simulink model "HANcoder_Olimexino_F3"  (R2018b)
settings: Solver=FixedStepDiscrete  StartTime=0.0  StopTime=2  FixedStep=0.01  RelTol=1e-3
PreLoadFcn:
  | librarySetup
  | eval([bdroot,'_startup']) %Calling [modelName]_startup.m
undefined symbols (not defined in the file or in its folder): A0, A1, A2, A3, A4, A5, CON2, CON3, CON4, D0, D14, D2, D24, D3, D5, D9, EXT, F3, HANtuneOverride, LED2, pwm, TIM2, TIM4, USB
libraries: HANcoder_STM32_Target x25, simulink x2
CloseFcn:
  | rtwprivate ssgencode ModelCloseRequest mytest
settings Model: Creator=Jason van Kolfschoten  LastModifiedBy=rickg
settings SolverCC: PositivePriorityOrder=on
settings DataIOCC: LimitDataPoints=on  SaveFormat=Array  SignalLoggingSaveFormat=ModelDataLogs  SaveOutput=off  SaveTime=off
settings OptimizationCC: BlockReduction=off  DefaultParameterBehavior=Inlined  DefaultUnderspecifiedDataType=single  InlineInvariantSignals=on  ExpressionDepthLimit=2147483647  StateBitsets=on  DataBitsets=on  ZeroExternalMemoryAtStartup=off  ZeroInternalMemoryAtStartup=off  InitFltsAndDblsToZero=on  NoFixptDivByZeroProtection=on  EfficientFloat2IntCast=on  LifeSpan=inf
settings DebuggingCC: SaveWithDisabledLinksMsg=none  SaveWithParameterizedLinksMsg=none  CheckSSInitialOutputMsg=off  UnderspecifiedInitializationDetection=Classic  MergeDetectMultiDrivingBlocksExec=none  SignalResolutionControl=TryResolveAll  SolverPrmCheckMsg=warning  InheritedTsInSrcMsg=none  MultiTaskDSMMsg=warning  MultiTaskCondExecSysMsg=none  ParameterPrecisionLossMsg=none  FcnCallInpInsideContextMsg=warning  StateNameClashWarn=warning  SFUnexpectedBacktrackingDiag=warning  SFNoUnconditionalDefaultTransitionDiag=warning  SFExecutionAtInitializationDiag=none
settings HardwareCC: ProdBitPerPointer=32  ProdBitPerSizeT=32  ProdBitPerPtrDiffT=32  ProdLargestAtomicInteger=Long  ProdLargestAtomicFloat=Double  ProdWordSize=32  ProdHWDeviceType=ARM Compatible->ARM Cortex  TargetEndianess=LittleEndian  TargetHWDeviceType=Infineon->TriCore
settings ModelReferenceCC: PropagateSignalLabelsOutOfModel=off
settings SFSimCC: SimUseLocalCustomCode=off  MATLABDynamicMemAlloc=off
settings RTWCC: SystemTargetFile=ert.tlc  MakeCommand=make_rtw SHELL= HANcoder_PORTABLE=1 HANcoder_BOOTLOADER=1  TemplateMakefile=Olimexino_STM32_F3_gcc.tmf  Description=Real-Time Workshop Embedded Coder (no auto configuration)  RTWUseLocalCustomCode=off
settings CodeAppCC: ForceParamTrailComments=on  IgnoreCustomStorageClasses=off  SimulinkDataObjDesc=on  CustomSymbolStrGlobalVar=rt$N$M  CustomSymbolStrType=$N$M  CustomSymbolStrFcn=$N$M$F  CustomSymbolStrMacro=$N$M  InsertBlockDesc=on  StateflowObjectComments=on  InternalIdentifier=Classic
settings ERTTargetCC: TargetFcnLib=ansi_tfl_tmw.mat  MultiwordLength=2048  IncludeMdlTerminateFcn=off  SuppressErrorStatus=on  SupportNonFinite=off  GenerateASAP2=on  InlinedParameterPlacement=NonHierarchical  ERTCustomFileTemplate=example_file_process.tlc  ConvertIfToSwitch=off  SuppressUnreachableDefaultCases=off
settings ConfigComp: CovMetricSettings=dw  CovHtmlReporting=on  CovSaveCumulativeToWorkspaceVar=on  CovSaveSingleToWorkspaceVar=on  CovExternalEMLEnable=off  CovSFcnEnable=off  DVMaxProcessTime=600  DVDisplayUnsatisfiableObjectives=on  DVAutomaticStubbing=off  DVSubSystemToStub=7.76600366011452e-316  DVParameterNames=7.76600366011452e-316  DVParameterConstraints=7.76600366011452e-316  DVParameterUseInAnalysis=7.76600366011452e-316  DVModelCoverageObjectives=MCDC  DVMaxTestCaseSteps=500  DVTestSuiteOptimization=CombinedObjectives  DVDetectActiveLogic=on  DVSaveHarnessModel=on

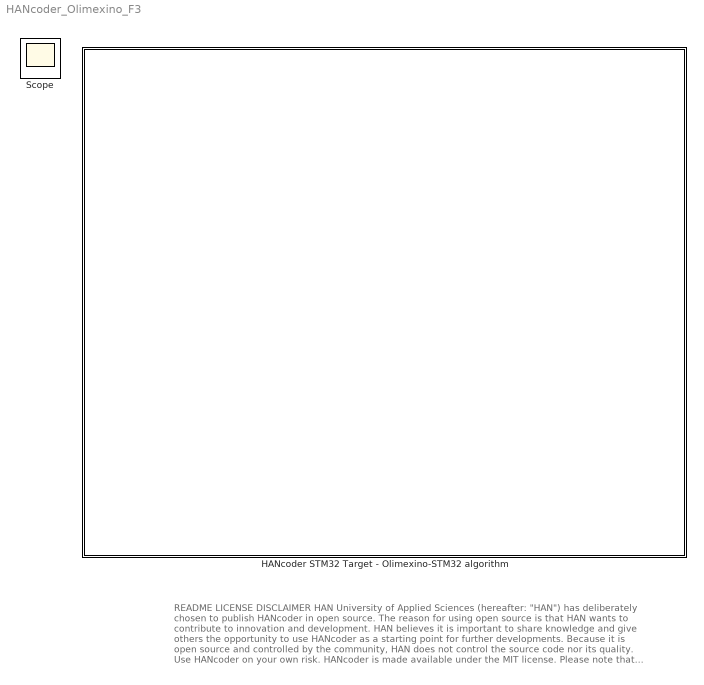
== system HANcoder_Olimexino_F3 ==
  note: README
      |
      | LICENSE
      |
      | DISCLAIMER
      |
      | HAN University of Applied Sciences (hereafter: "HAN") has deliberately chosen
      | to publish HANcoder in open source. The reason for using open source is that
      | HAN wants to contribute to innovation and development. HAN believes it is
      | important to share knowledge and give others the opportunity to use HANcoder
      | as a starting point for further developments. Because it is open source and
      | controlled by the community, HAN does not control the source code nor its
      | quality. Use HANcoder on your own risk. HANcoder is made available under the
      | MIT license. Please note that this license contains an exclusion of liability.
  HANcoder STM32 Target - Olimexino-STM32 algorithm : Subsystem  mask(TopLevelSubsystem){}
      mask Display: image(imread('Olimexino_STM32_HAN.jpg'))
  Scope : Scope

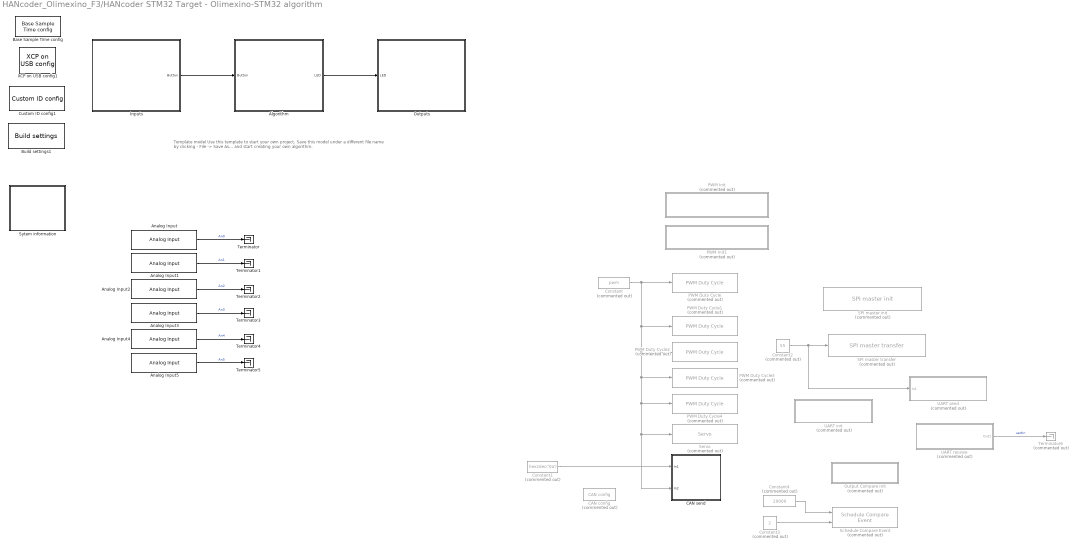
== system HANcoder_Olimexino_F3/HANcoder STM32 Target - Olimexino-STM32 algorithm ==
  note: Template model
      | Use this template to start your own project. Save this model
      | under a different file name by clicking - File -> Save As... and
      | start creating your own algorithm.
  Algorithm : Subsystem
  Analog Input : HANcoder_STM32_Target/Olimexino STM32 F3/Analog Inputs/Analog Input  Tag=HANcoder_TARGET_STM32_F3_Olimexino  pinID=CON2 - A0  tsamp=-1  filtered=off
      settings: SourceProductName=HANcoder STM32 Target
  Analog Input1 : HANcoder_STM32_Target/Olimexino STM32 F3/Analog Inputs/Analog Input  Tag=HANcoder_TARGET_STM32_F3_Olimexino  pinID=CON2 - A1  tsamp=-1  filtered=off
      settings: SourceProductName=HANcoder STM32 Target
  Analog Input2 : HANcoder_STM32_Target/Olimexino STM32 F3/Analog Inputs/Analog Input  Tag=HANcoder_TARGET_STM32_F3_Olimexino  pinID=CON2 - A2  tsamp=-1  filtered=off
      settings: SourceProductName=HANcoder STM32 Target
  Analog Input3 : HANcoder_STM32_Target/Olimexino STM32 F3/Analog Inputs/Analog Input  Tag=HANcoder_TARGET_STM32_F3_Olimexino  pinID=CON2 - A3  tsamp=-1  filtered=off
      settings: SourceProductName=HANcoder STM32 Target
  Analog Input4 : HANcoder_STM32_Target/Olimexino STM32 F3/Analog Inputs/Analog Input  Tag=HANcoder_TARGET_STM32_F3_Olimexino  pinID=CON2 - A4  tsamp=-1  filtered=off
      settings: SourceProductName=HANcoder STM32 Target
  Analog Input5 : HANcoder_STM32_Target/Olimexino STM32 F3/Analog Inputs/Analog Input  Tag=HANcoder_TARGET_STM32_F3_Olimexino  pinID=CON2 - A5  tsamp=-1  filtered=off
      settings: SourceProductName=HANcoder STM32 Target
  Base Sample Time config : HANcoder_STM32_Target/Olimexino STM32 F3/System Config/Base Sample Time config  Tag=HANcoder_TARGET_STM32_F3_Olimexino  Description=HANcoder Target STM32-Olimexino blockset version 1.2  baseSampleTime=10  extraStack=25
      settings: SourceProductName=HANcoder STM32 Target
  Build settings1 : HANcoder_STM32_Target/Olimexino STM32 F3/System Config/Build settings  Tag=HANcoder_TARGET_STM32_F3_Olimexino  AutoASAP2add=on  AutoFlash=USB-F3
      settings: SourceProductName=HANcoder STM32 Target
  CAN config : HANcoder_STM32_Target/Olimexino STM32 F3/System Config/CAN config  Tag=HANcoder_TARGET_STM32_F3_Olimexino  Commented=on  canBus1=on  baudRate1=250  rxMask1=hex2dec('00000000')  rxCode1=hex2dec('00000000')  rxMode1=Receive only 11-bit message identifiers  txBufSize1=32  evBufSize1=8
      settings: SourceProductName=HANcoder STM32 Target
  CAN send : Subsystem  Tag=HANcoder_TARGET_STM32_F3_Olimexino  AncestorBlock=HANcoder_STM32_Target/Olimexino STM32 F3/CAN/CAN/CAN send  mask(CAN send){canBus=CAN 1, frameType=Standard (11 bit), inputNumber=1, dataType=uint16, byteOrder=on, tsamp=0.1}
      mask prompts: canBus "CAN channel"; frameType "Identifier type"; inputNumber "Input ports"; dataType "Input datatype"; byteOrder "Byte order: Checked = MSB first, unchecked = LSB first."; tsamp "Sample time"
      mask help:
      | Function
      | ==========
      | Send a message on the CAN channel.
      |
      | Parameters
      | ==========
      | CAN channel:           The CAN channel to send the message on.
      | Identifier type:         normal or extended ID's
      | Input ports:              The amount of input ports
      | Input datatype:        The datatype of the input ports
      | Byte order:               Select MSB or LSB first
      | Sample time:            -1 or divisible by base sample time [seconds]
      |
      | Input
      | ==========
      | Port 1:                   CAN ID(uint32) in hexadecimal ie: hex2dec('0a')
      | Port 2..9                CAN message data
      mask init:
      | sfcn_can_send_mcb(canBus, frameType, inputNumber, dataType, byteOrder)
      settings: MoveFcn=drawLogos
      mask Help: web('sfcn_can_send.html');
      mask TypeOptions canBus: CAN 1
      mask TypeOptions frameType: Standard (11 bit) | Extended (29 bit)
      mask TypeOptions dataType: int8 | uint8 | int16 | uint16 | int32 | uint32 | boolean
      mask Display:
      | fprintf('Send on\nCAN %x', canBus);
      | port_label('input', 1, 'ID');patch([89 108 107 88],[2 6 10 6],[0.89804 0 0.33725]);
  Constant : Constant  Commented=on  Value=pwm  OutDataTypeStr=uint16
  Constant1 : Constant  Commented=on  Value=hex2dec('0a')  OutDataTypeStr=uint32
  Constant2 : Constant  Commented=on  Value=55  OutDataTypeStr=uint8
  Constant3 : Constant  Commented=on  Value=2  OutDataTypeStr=uint8
  Constant4 : Constant  Commented=on  Value=20000  OutDataTypeStr=uint16
  Custom ID config1 : HANcoder_STM32_Target/Olimexino STM32 F3/System Config/Custom ID config  Tag=HANcoder_TARGET_STM32_F3_Olimexino  softID=softwareID  softNUM=1
      settings: SourceProductName=HANcoder STM32 Target
  Inputs : Subsystem
  Output Compare Init : Subsystem  Tag=HANcoder_TARGET_STM32_F3_Olimexino  Commented=on  AncestorBlock=HANcoder_STM32_Target/Olimexino STM32 F3/Timer Outputs/Output Compare Init  mask(Output Compare Init){moduleID=TIM2: D2 & D3 & D1 & D0, frequency=2000000, enableIRQoutput=off}
      mask prompts: moduleID "Timer module"; frequency "Frequency (free running counter) [Hz]"; enableIRQoutput "Enable IRQ output"
      mask help:
      | Function
      | ========
      | Initializes the timer module to allow output compare functionality on the
      | module's channels.
      |
      | Parameters
      | ==========
      | Timer Module:
      |   Selects the timer module.
      |
      | Frequency:
      |   Frequency at which the 16-bit free running counter counts.
      |
      | Enable IRQ output
      |   Controls whether or not the IRQ output is available.
      |
      | Outport
      | =======
      | IRQ
      |   Allows connection of a function call subsystem for the free running
      |   counter overflow event.
      mask init:
      | moduleIDInfoStr = sfcn_timeout_init_mcb(1, moduleID, frequency, enableIRQoutput);
      settings: CopyFcn=sfcn_timeout_init_chk();  MoveFcn=drawLogos
      mask Help: web('sfcn_timeout_init.html');
      mask TypeOptions moduleID: TIM1: D6 & D7 & D8 & n/a | TIM2: D2 & D3 & D1 & D0 | TIM3: D35 & D36 & D37 & n/a | TIM4: D5 & D9 & D14 & D24
      mask Callback moduleID: sfcn_timeout_init_chk();
      mask Display: fprintf('Output Compare Init\n%s', moduleIDInfoStr);patch([129 148 147 128],[2 6 10 6],[0.89804 0 0.33725]);
  Outputs : Subsystem
  PWM Duty Cycle : HANcoder_STM32_Target/Olimexino STM32 F3/PWM Outputs/PWM Duty Cycle  Tag=HANcoder_TARGET_STM32_F3_Olimexino  Commented=on  pinID=TIM2 - CON3 - D0  tsamp=-1
      settings: SourceProductName=HANcoder STM32 Target
  PWM Duty Cycle1 : HANcoder_STM32_Target/Olimexino STM32 F3/PWM Outputs/PWM Duty Cycle  Tag=HANcoder_TARGET_STM32_F3_Olimexino  Commented=on  pinID=TIM4 - CON3 - D5  tsamp=-1
      settings: SourceProductName=HANcoder STM32 Target
  PWM Duty Cycle2 : HANcoder_STM32_Target/Olimexino STM32 F3/PWM Outputs/PWM Duty Cycle  Tag=HANcoder_TARGET_STM32_F3_Olimexino  Commented=on  pinID=TIM4 - CON4 - D9  tsamp=-1
      settings: SourceProductName=HANcoder STM32 Target
  PWM Duty Cycle3 : HANcoder_STM32_Target/Olimexino STM32 F3/PWM Outputs/PWM Duty Cycle  Tag=HANcoder_TARGET_STM32_F3_Olimexino  Commented=on  pinID=TIM4 - CON4 - D14  tsamp=-1
      settings: SourceProductName=HANcoder STM32 Target
  PWM Duty Cycle4 : HANcoder_STM32_Target/Olimexino STM32 F3/PWM Outputs/PWM Duty Cycle  Tag=HANcoder_TARGET_STM32_F3_Olimexino  Commented=on  pinID=TIM4 - EXT - D24  tsamp=-1
      settings: SourceProductName=HANcoder STM32 Target
  PWM Init : Subsystem  Tag=HANcoder_TARGET_STM32_F3_Olimexino  Commented=on  AncestorBlock=HANcoder_STM32_Target/Olimexino STM32 F3/PWM Outputs/PWM Init  mask(Pulse Width Modulation Initialization){moduleID=TIM2: D2 & D3 & n/a & D0, frequency=5022, alignment=Edge aligned, enableIRQoutput=off, ch1On=off, ch1Pol=Active high, ch1Inv=off, ch2On=off, ch2Pol=Active high, ch2Inv=off, ch3On=off, ch3Pol=Active high, ch3Inv=off, ch4On=on, ch4Pol=Active high, ch4Inv=off}
      mask prompts: moduleID "PWM module"; frequency "Signal frequency [Hz]"; alignment "Signal alignment"; enableIRQoutput "Enable IRQ output"; ch1On "Generate PWM signal on channel 1"; ch1Pol "Select signal polarity"; ch1Inv "Enable inverted signal on additional output pin"; ch2On "Generate PWM signal on channel 2"; ch2Pol "Select signal polarity"; ch2Inv "Enable inverted signal on additional output pin"; ch3On "Generate PWM signal on channel 3"; ch3Pol "Select signal polarity"; ch3Inv "Enable inverted signal on additional output pin"; ch4On "Generate PWM signal on channel 4"; ch4Pol "Select signal polarity"; ch4Inv "Enable inverted signal on additional output pin"
      mask help:
      | Function
      | ========
      | A 'PWM Init' block configures one of the STM32 timer modules for PWM
      | functionality, allowing a PWM signal to be generated on up to 4 timer
      | channels and their associated output pins.
      |
      | Parameters
      | ==========
      | General - PWM module:
      |   Select the PWM module to use. The name in the combo box contains
      |   information about which pins on the target belong to this timer module.
      |   Also the first pin corresponds with the first channel and so on:
      |   TIMx: Ch1 & Ch2 & Ch3...
      |
      | General - Signal frequency:
      |   Determines the signal frequency in Hz. If you click 'Apply' after entering
      |   the desired frequency it will automatically be adjusted to the closest
      |   supported value.
      |
      | General - Signal Aligment:
      |   Determines the aligment of the signal. It can either be edge aligned or
      |   center aligned.
      |
      | General - Enable IRQ output
      |   Controls whether or not the IRQ output is available.
      |
      | Channel x - Generate PWM signal on channel x:
      |   Enable to configure the channel for PWM functionality so that the PWM signal
      |   is outputted on the channel's associated microcontroller pin.
      |
      | Channel x - Signal polarity:
      |   Selects the polarity of the signal.
      |
      | Channel x - Enable inverted signal on additional output pin:
      |   When enabled, a second PWM signal will be generated on an additional
      |   microcontroller pin where the signal is an exact inversion of the first signal.
      mask init:
      | moduleIDInfoStr = sfcn_pwmout_init_mcb(1, moduleID, frequency, alignment, enableIRQoutput, ch1On, ch2On, ch3On, ch4On, ch1Pol, ch2Pol, ch3Pol, ch4Pol, ch1Inv, ch2Inv, ch3Inv, ch4Inv);
      settings: CopyFcn=sfcn_pwmout_init_chk();  MoveFcn=drawLogos
      mask Help: web('sfcn_pwmout_init.html');
      mask TypeOptions moduleID: TIM1: D6 & D7 & D8 & n/a + N-channels D32 & D33 & D34  | TIM2: D2 & D3 & n/a & D0 | TIM3: D35 & D36 & D37 & n/a | TIM4: D5 & D9 & D14 & D24
      mask Callback moduleID: sfcn_pwmout_init_chk();
      mask TypeOptions alignment: Edge aligned | Center aligned
      mask TypeOptions ch1Pol: Active high | Active low
      mask TypeOptions ch2Pol: Active high | Active low
      mask TypeOptions ch3Pol: Active high | Active low
      mask TypeOptions ch4Pol: Active high | Active low
      mask Display: fprintf('PWM Init\n%s', moduleIDInfoStr);patch([214 233 232 213],[2 6 10 6],[0.89804 0 0.33725]);
  PWM Init1 : Subsystem  Tag=HANcoder_TARGET_STM32_F3_Olimexino  Commented=on  AncestorBlock=HANcoder_STM32_Target/Olimexino STM32 F3/PWM Outputs/PWM Init  mask(Pulse Width Modulation Initialization){moduleID=TIM4: D5 & D9 & D14 & D24, frequency=5022, alignment=Edge aligned, enableIRQoutput=off, ch1On=on, ch1Pol=Active high, ch1Inv=off, ch2On=on, ch2Pol=Active high, ch2Inv=off, ch3On=off, ch3Pol=Active high, ch3Inv=off, ch4On=off, ch4Pol=Active high, ch4Inv=off}
      mask prompts: moduleID "PWM module"; frequency "Signal frequency [Hz]"; alignment "Signal alignment"; enableIRQoutput "Enable IRQ output"; ch1On "Generate PWM signal on channel 1"; ch1Pol "Select signal polarity"; ch1Inv "Enable inverted signal on additional output pin"; ch2On "Generate PWM signal on channel 2"; ch2Pol "Select signal polarity"; ch2Inv "Enable inverted signal on additional output pin"; ch3On "Generate PWM signal on channel 3"; ch3Pol "Select signal polarity"; ch3Inv "Enable inverted signal on additional output pin"; ch4On "Generate PWM signal on channel 4"; ch4Pol "Select signal polarity"; ch4Inv "Enable inverted signal on additional output pin"
      mask help:
      | Function
      | ========
      | A 'PWM Init' block configures one of the STM32 timer modules for PWM
      | functionality, allowing a PWM signal to be generated on up to 4 timer
      | channels and their associated output pins.
      |
      | Parameters
      | ==========
      | General - PWM module:
      |   Select the PWM module to use. The name in the combo box contains
      |   information about which pins on the target belong to this timer module.
      |   Also the first pin corresponds with the first channel and so on:
      |   TIMx: Ch1 & Ch2 & Ch3...
      |
      | General - Signal frequency:
      |   Determines the signal frequency in Hz. If you click 'Apply' after entering
      |   the desired frequency it will automatically be adjusted to the closest
      |   supported value.
      |
      | General - Signal Aligment:
      |   Determines the aligment of the signal. It can either be edge aligned or
      |   center aligned.
      |
      | General - Enable IRQ output
      |   Controls whether or not the IRQ output is available.
      |
      | Channel x - Generate PWM signal on channel x:
      |   Enable to configure the channel for PWM functionality so that the PWM signal
      |   is outputted on the channel's associated microcontroller pin.
      |
      | Channel x - Signal polarity:
      |   Selects the polarity of the signal.
      |
      | Channel x - Enable inverted signal on additional output pin:
      |   When enabled, a second PWM signal will be generated on an additional
      |   microcontroller pin where the signal is an exact inversion of the first signal.
      mask init:
      | moduleIDInfoStr = sfcn_pwmout_init_mcb(1, moduleID, frequency, alignment, enableIRQoutput, ch1On, ch2On, ch3On, ch4On, ch1Pol, ch2Pol, ch3Pol, ch4Pol, ch1Inv, ch2Inv, ch3Inv, ch4Inv);
      settings: CopyFcn=sfcn_pwmout_init_chk();  MoveFcn=drawLogos
      mask Help: web('sfcn_pwmout_init.html');
      mask TypeOptions moduleID: TIM1: D6 & D7 & D8 & n/a + N-channels D32 & D33 & D34  | TIM2: D2 & D3 & n/a & D0 | TIM3: D35 & D36 & D37 & n/a | TIM4: D5 & D9 & D14 & D24
      mask Callback moduleID: sfcn_pwmout_init_chk();
      mask TypeOptions alignment: Edge aligned | Center aligned
      mask TypeOptions ch1Pol: Active high | Active low
      mask TypeOptions ch2Pol: Active high | Active low
      mask TypeOptions ch3Pol: Active high | Active low
      mask TypeOptions ch4Pol: Active high | Active low
      mask Display: fprintf('PWM Init\n%s', moduleIDInfoStr);patch([214 233 232 213],[2 6 10 6],[0.89804 0 0.33725]);
  SPI master init : HANcoder_STM32_Target/Olimexino STM32 F3/SPI/SPI master init  Tag=HANcoder_TARGET_STM32_F3_Olimexino  Commented=on  channel=SPI1: D13 & D12 & D11  speed=9000 kHz  polarity=Idle low  phase=Sample bit on 1st clock edge
      settings: SourceProductName=HANcoder STM32 Target
  SPI master transfer : HANcoder_STM32_Target/Olimexino STM32 F3/SPI/SPI master transfer  Tag=HANcoder_TARGET_STM32_F3_Olimexino  Priority=1  Commented=on  channel=SPI1: D13 & D12 & D11  useSS=off  SSpin=CON2 - A0  SSenable=on  SSdisable=on  delayCycles=0  userPriority=1  tsamp=-1
      settings: SourceProductName=HANcoder STM32 Target
  Schedule Compare Event : HANcoder_STM32_Target/Olimexino STM32 F3/Timer Outputs/Schedule Compare Event  Tag=HANcoder_TARGET_STM32_F3_Olimexino  Commented=on  pin=TIM2: CON3 - D3  tsamp=-1
      settings: SourceProductName=HANcoder STM32 Target
  Servo : HANcoder_STM32_Target/Olimexino STM32 F3/Servo/Servo  Tag=HANcoder_TARGET_STM32_F3_Olimexino  Commented=on  pinID=TIM2 - CON3 - D2  lowerLimit=1000  upperLimit=2000  tsamp=-1
      settings: SourceProductName=HANcoder STM32 Target
  Sytem information : Subsystem
  Terminator{,1..5} (6 alike) : Terminator
  Terminator6 : Terminator  Commented=on
  UART init : Subsystem  Tag=HANcoder_TARGET_STM32_F3_Olimexino  Commented=on  AncestorBlock=HANcoder_STM32_Target/Olimexino STM32 F3/UART/UART init  mask(UART init){channel=UART1: D7 & D8, baudrate=19200, databits=8, parity=none, stopbits=1, txbufsize=32, rxbufsize=32, useStatusOut=off}
      mask prompts: baudrate "Baudrate (bit/s)"; txbufsize "Transmit buffer size"; rxbufsize "Receive buffer size"; useStatusOut "Use status output"
      mask help:
      | Function
      | ==========
      | Initialized a UART channel.
      |
      | Parameters per channel
      | ======================
      | - Select channel
      | - Select baudrate
      | - Select number of databits
      | - Select parity
      | - Select number of stopbits
      | - Configure the size of the transmit buffer
      | - Configure the size of the reception buffer
      | - Enable/disable the status output port
      mask init:
      | uartChannelInfoStr = sfcn_uart_init_mcb(1, channel, baudrate, databits, parity, stopbits, txbufsize, rxbufsize, useStatusOut);
      settings: CopyFcn=sfcn_uart_init_chk();  MoveFcn=drawLogos
      mask Help: web('sfcn_uart_init.html')
      mask TypeOptions channel: UART1: D7 & D8 | UART2: D1 & D0 | UART3: D29 & D30
      mask Callback channel: sfcn_uart_init_chk();
      mask TypeOptions baudrate: 300 | 600 | 1200 | 2400 | 4800 | 9600 | 19200 | 38400 | 57600 | 115200
      mask TypeOptions databits: 8 | 9
      mask TypeOptions parity: none | even | odd
      mask TypeOptions stopbits: 1 | 2
      mask Display: fprintf('UART init\n%s', uartChannelInfoStr);patch([155 174 173 154],[2 6 10 6],[0.89804 0 0.33725]);
  UART receive : Subsystem  Tag=HANcoder_TARGET_STM32_F3_Olimexino  Commented=on  AncestorBlock=HANcoder_STM32_Target/Olimexino STM32 F3/UART/UART receive  mask(UART receive){channel=UART1: D7 & D8, useStatusOut=off, tsamp=-1}
      mask prompts: useStatusOut "Use status outport"; tsamp "Sample time"
      mask help:
      | Function
      | ==========
      | Reads a byte from the UART reception buffer.
      |
      | Parameters per channel
      | ======================
      | - Select channel
      | - Select if the status output should be enabled.
      |
      | Outputs
      | =======
      | - The value of the receive byte.
      | - When the status output is 0, the reception buffer was empty.
      mask init:
      | uartChannelInfoStr = sfcn_uart_receive_mcb(1, channel, useStatusOut);
      settings: MoveFcn=drawLogos
      mask Help: web('sfcn_uart_receive.html')
      mask TypeOptions channel: UART1: D7 & D8 | UART2: D1 & D0 | UART3: D29 & D30
      mask Display: fprintf('UART receive\n%s', uartChannelInfoStr);patch([154 173 172 153],[2 6 10 6],[0.89804 0 0.33725]);
  UART send : Subsystem  Tag=HANcoder_TARGET_STM32_F3_Olimexino  Commented=on  AncestorBlock=HANcoder_STM32_Target/Olimexino STM32 F3/UART/UART send  mask(UART send){channel=UART1: D7 & D8, useStatusOut=off, tsamp=-1}
      mask prompts: useStatusOut "Use status outport"; tsamp "Sample time"
      mask help:
      | Function
      | ==========
      | Transmits a byte on the UART communication interface.
      |
      | Parameters per channel
      | ======================
      | - Select channel
      | - Select if the status output should be enabled.
      |
      | Inputs
      | ======
      | - The byte to send
      |
      | Outputs
      | =======
      | - When the status output is 0, the byte could not be transmitted. Probably
      |   because the transmit buffer was configured too small.
      mask init:
      | uartChannelInfoStr = sfcn_uart_send_mcb(1, channel, useStatusOut);
      settings: MoveFcn=drawLogos
      mask Help: web('sfcn_uart_send.html')
      mask TypeOptions channel: UART1: D7 & D8 | UART2: D1 & D0 | UART3: D29 & D30
      mask Display: fprintf('UART send\n%s', uartChannelInfoStr);patch([154 173 172 153],[2 6 10 6],[0.89804 0 0.33725]);
  XCP on USB config1 : HANcoder_STM32_Target/Olimexino STM32 F3/System Config/XCP on USB config  Tag=HANcoder_TARGET_STM32_F3_Olimexino
      settings: SourceProductName=HANcoder STM32 Target
  wires:
  Inputs/1(Button) -> Algorithm/1(Button)
  Algorithm/1(LED) -> Outputs/1(LED)
  Analog Input/1 -> Terminator/1  "An0"
  Analog Input1/1 -> Terminator1/1  "An1"
  Analog Input2/1 -> Terminator2/1  "An2"
  Analog Input3/1 -> Terminator3/1  "An3"
  Analog Input4/1 -> Terminator4/1  "An4"
  Analog Input5/1 -> Terminator5/1  "An5"
  Constant/1 -> PWM Duty Cycle1/1, PWM Duty Cycle2/1, PWM Duty Cycle3/1, Servo/1, CAN send/2(In2), PWM Duty Cycle4/1, PWM Duty Cycle/1
  Constant1/1 -> CAN send/1(In1)
  Constant2/1 -> UART send/1(In1), SPI master transfer/1
  UART receive/1(Out1) -> Terminator6/1  "uartin"
  Constant3/1 -> Schedule Compare Event/2
  Constant4/1 -> Schedule Compare Event/1

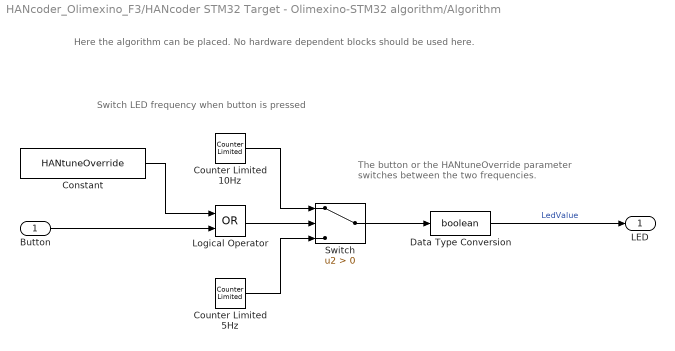
== system HANcoder_Olimexino_F3/HANcoder STM32 Target - Olimexino-STM32 algorithm/Algorithm ==
  note: The button or the HANtuneOverride parameter
      | switches between the two frequencies.
  note: Switch LED frequency when button is pressed
  note: Here the algorithm can be placed. No hardware dependent blocks should be used here.
  Button : Inport
  Constant : Constant  Value=HANtuneOverride  OutDataTypeStr=boolean
  Counter Limited 10Hz : simulink/Sources/Counter Limited  uplimit=1  tsamp=0.1
  Counter Limited 5Hz : simulink/Sources/Counter Limited  uplimit=1  tsamp=0.2
  Data Type Conversion : DataTypeConversion  OutDataTypeStr=boolean
  Logical Operator : Logic  Operator=OR  AllPortsSameDT=off  OutDataTypeStr=boolean
  Switch : Switch  Criteria=u2 > Threshold
  LED : Outport
  wires:
  Data Type Conversion/1 -> LED/1  "LedValue"
  Counter Limited 5Hz/1 -> Switch/3
  Switch/1 -> Data Type Conversion/1
  Button/1 -> Logical Operator/2
  Logical Operator/1 -> Switch/2
  Constant/1 -> Logical Operator/1
  Counter Limited 10Hz/1 -> Switch/1

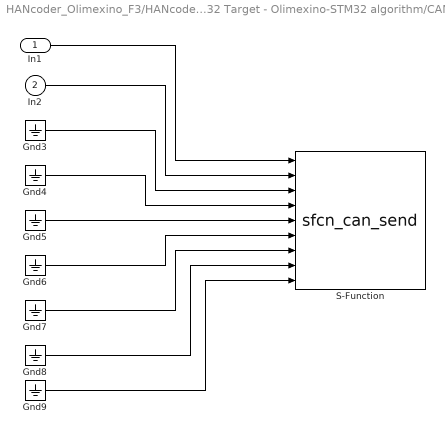
== system HANcoder_Olimexino_F3/HANcoder STM32 Target - Olimexino-STM32 algorithm/CAN send ==
  In1 : Inport
  In2 : Inport  Port=2
  Gnd{3..9} (7 alike) : Ground
  S-Function : M-S-Function  FunctionName=sfcn_can_send  Parameters=tsamp, canBus, frameType, inputNumber, dataType, byteOrder
  wires:
  Gnd9/1 -> S-Function/9
  Gnd8/1 -> S-Function/8
  Gnd7/1 -> S-Function/7
  Gnd6/1 -> S-Function/6
  Gnd5/1 -> S-Function/5
  Gnd4/1 -> S-Function/4
  Gnd3/1 -> S-Function/3
  In2/1 -> S-Function/2
  In1/1 -> S-Function/1

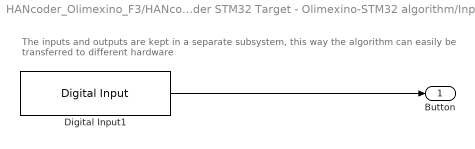
== system HANcoder_Olimexino_F3/HANcoder STM32 Target - Olimexino-STM32 algorithm/Inputs ==
  note: The inputs and outputs are kept in a separate subsystem, this way the algorithm can easily be transferred to different hardware
  Digital Input1 : HANcoder_STM32_Target/Olimexino STM32 F3/Digital Inputs/Digital Input  Tag=HANcoder_TARGET_STM32_F3_Olimexino  pinID=Pushbutton - BUT/BOOT0 - 5V Tolerant  config=Pulldown  tsamp=-1
      settings: SourceProductName=HANcoder STM32 Target
  Button : Outport
  wires:
  Digital Input1/1 -> Button/1

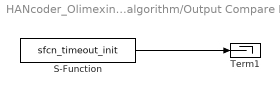
== system HANcoder_Olimexino_F3/HANcoder STM32 Target - Olimexino-STM32 algorithm/Output Compare Init ==
  S-Function : S-Function  FunctionName=sfcn_timeout_init  SFunctionDeploymentMode=off  EnableBusSupport=off
  Term1 : Terminator
  wires:
  S-Function/1 -> Term1/1

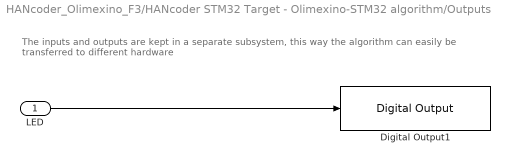
== system HANcoder_Olimexino_F3/HANcoder STM32 Target - Olimexino-STM32 algorithm/Outputs ==
  note: The inputs and outputs are kept in a separate subsystem, this way the algorithm can easily be transferred to different hardware
  LED : Inport
  Digital Output1 : HANcoder_STM32_Target/Olimexino STM32 F3/Digital Outputs/Digital Output  Tag=HANcoder_TARGET_STM32_F3_Olimexino  pinID=CON3 - D3/LED2  config=Push pull  tsamp=-1
      settings: SourceProductName=HANcoder STM32 Target
  wires:
  LED/1 -> Digital Output1/1

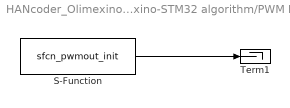
== system HANcoder_Olimexino_F3/HANcoder STM32 Target - Olimexino-STM32 algorithm/PWM Init ==
  S-Function : S-Function  FunctionName=sfcn_pwmout_init  SFunctionDeploymentMode=off  EnableBusSupport=off
  Term1 : Terminator
  wires:
  S-Function/1 -> Term1/1

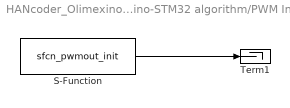
== system HANcoder_Olimexino_F3/HANcoder STM32 Target - Olimexino-STM32 algorithm/PWM Init1 ==
  S-Function : S-Function  FunctionName=sfcn_pwmout_init  SFunctionDeploymentMode=off  EnableBusSupport=off
  Term1 : Terminator
  wires:
  S-Function/1 -> Term1/1

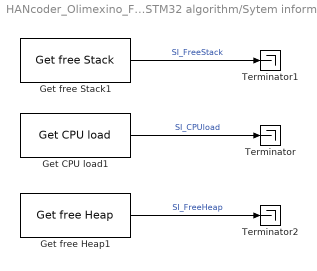
== system HANcoder_Olimexino_F3/HANcoder STM32 Target - Olimexino-STM32 algorithm/Sytem information ==
  Get CPU load1 : HANcoder_STM32_Target/Olimexino STM32 F3/System Management/Get CPU load  Tag=HANcoder_TARGET_STM32_F3_Olimexino  mode=Current CPU load  tsamp=-1
      settings: SourceProductName=HANcoder STM32 Target
  Get free Heap1 : HANcoder_STM32_Target/Olimexino STM32 F3/System Management/Get free Heap  Tag=HANcoder_TARGET_STM32_F3_Olimexino  tsamp=-1
      settings: SourceProductName=HANcoder STM32 Target
  Get free Stack1 : HANcoder_STM32_Target/Olimexino STM32 F3/System Management/Get free Stack  Tag=HANcoder_TARGET_STM32_F3_Olimexino  taskIdx=Application Control Task  tsamp=-1
      settings: SourceProductName=HANcoder STM32 Target
  Terminator : Terminator
  Terminator1 : Terminator
  Terminator2 : Terminator
  wires:
  Get CPU load1/1 -> Terminator/1  "SI_CPUload"
  Get free Stack1/1 -> Terminator1/1  "SI_FreeStack"
  Get free Heap1/1 -> Terminator2/1  "SI_FreeHeap"

== system HANcoder_Olimexino_F3/HANcoder STM32 Target - Olimexino-STM32 algorithm/UART init ==
  Level-2 M-file S-Function : M-S-Function  FunctionName=sfcn_uart_init
  Term1 : Terminator
  wires:
  Level-2 M-file S-Function/1 -> Term1/1

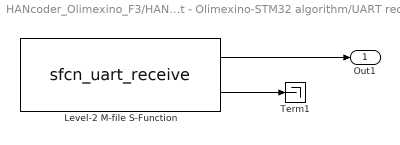
== system HANcoder_Olimexino_F3/HANcoder STM32 Target - Olimexino-STM32 algorithm/UART receive ==
  Level-2 M-file S-Function : M-S-Function  FunctionName=sfcn_uart_receive  Parameters=tsamp
  Term1 : Terminator
  Out1 : Outport
  wires:
  Level-2 M-file S-Function/1 -> Out1/1
  Level-2 M-file S-Function/2 -> Term1/1

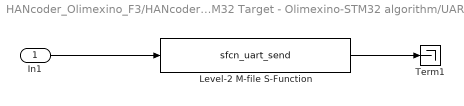
== system HANcoder_Olimexino_F3/HANcoder STM32 Target - Olimexino-STM32 algorithm/UART send ==
  In1 : Inport
  Level-2 M-file S-Function : M-S-Function  FunctionName=sfcn_uart_send  Parameters=tsamp
  Term1 : Terminator
  wires:
  Level-2 M-file S-Function/1 -> Term1/1
  In1/1 -> Level-2 M-file S-Function/1
